simulink model "pend"  (R2018b)
settings: Solver=ode45  StartTime=0.0  StopTime=1.4  RelTol=1e-6
values from neighbouring files (symbols this model uses):
  g = 9.81    [plate_pend.m]
  J_zz = m_plate*(Lx^2+Ly^2)/3    (= 2.1087)    [plate_pend.m]
  Lx = 0.5    [parameters.m]    (also in plate_pend.m = 0.6)
  Ly = 0.3    [parameters.m]    (also in plate_pend.m)
  m_plate = rho*h*Lx*Ly    (= 9.36)    [parameters.m]    (also in plate_pend.m = 14.058)
libraries: cstblocks x1
settings Model: Creator=a.brugnoli  LastModifiedBy=a.brugnoli

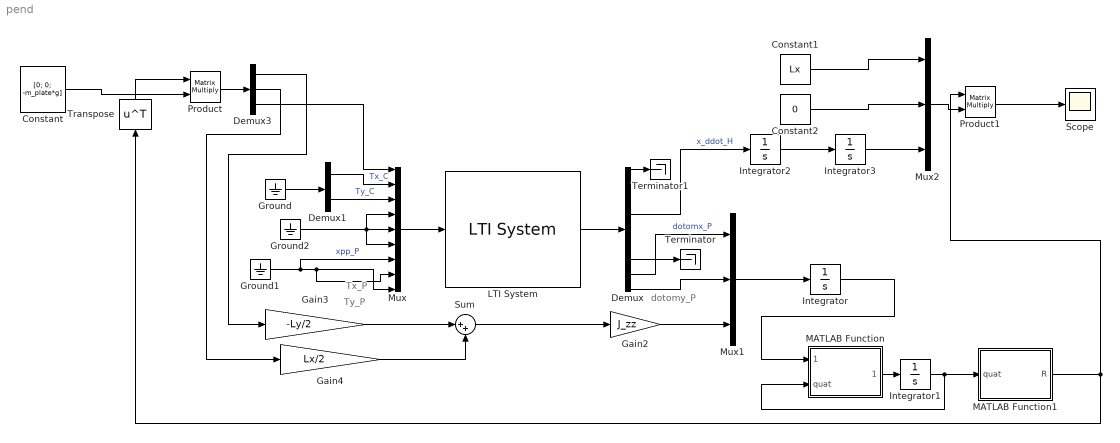
== system pend ==
  note: dotomy_P
  note: Ty_P
  note: Tx_P
  Constant : Constant  Value=[0; 0; -m_plate*g]  VectorParams1D=off
  Constant1 : Constant  Value=Lx
  Constant2 : Constant  Value=0
  Demux : Demux  Outputs=9
  Demux1 : Demux  Outputs=2
  Demux3 : Demux  Outputs=3
  Gain2 : Gain  Gain=J_zz
  Gain3 : Gain  Gain=-Ly/2
  Gain4 : Gain  Gain=Lx/2
  Ground : Ground
  Ground1 : Ground
  Ground2 : Ground
  Integrator : Integrator
  Integrator1 : Integrator  InitialCondition=[1, 0, 0, 0]
  Integrator2 : Integrator
  Integrator3 : Integrator
  LTI System : cstblocks/LTI System  sys=plate_pendulum  IC=[]
  MATLAB Function : MATLAB Function  TreatAsAtomicUnit=on
  MATLAB Function1 : MATLAB Function  TreatAsAtomicUnit=on
  Mux : Mux  Inputs=9
  Mux1 : Mux  Inputs=3
  Mux2 : Mux  Inputs=3
  Product : Product  Multiplication=Matrix(*)
  Product1 : Product  Multiplication=Matrix(*)
  Scope : Scope
  Sum : Sum  Inputs=|++
  Terminator : Terminator
  Terminator1 : Terminator
  Transpose : Math  Operator=transpose  SaturateOnIntegerOverflow=on
  wires:
  LTI System/1 -> Demux/1
  Mux/1 -> LTI System/1
  Ground/1 -> Demux1/1
  Demux1/2 -> Mux/3  "Ty_C"
  Demux1/1 -> Mux/2  "Tx_C"
  Gain2/1 -> Mux1/3
  Ground1/1 -> Mux/9, Mux/8, Mux/7  "xpp_P"
  Demux3/3 -> Mux/1
  Demux3/2 -> Gain4/1
  Demux3/1 -> Gain3/1
  Mux1/1 -> Integrator/1
  Integrator/1 -> MATLAB Function/1(omega)
  MATLAB Function/1(dt_quat) -> Integrator1/1
  Integrator1/1 -> MATLAB Function1/1(quat), MATLAB Function/2(quat)
  MATLAB Function1/1(R) -> Product1/1, Transpose/1
  Transpose/1 -> Product/1
  Constant/1 -> Product/2
  Product/1 -> Demux3/1
  Gain4/1 -> Sum/2
  Gain3/1 -> Sum/1
  Sum/1 -> Gain2/1
  Demux/9 -> Mux1/2
  Demux/8 -> Mux1/1  "dotomx_P"
  Demux/7 -> Terminator/1
  Demux/4 -> Integrator2/1  "x_ddot_H"
  Ground2/1 -> Mux/6, Mux/4, Mux/5
  Integrator2/1 -> Integrator3/1
  Integrator3/1 -> Mux2/3
  Constant2/1 -> Mux2/2
  Constant1/1 -> Mux2/1
  Mux2/1 -> Product1/2
  Product1/1 -> Scope/1
  Demux/1 -> Terminator1/1

== matlab function pend/MATLAB Function1 ==
  data: R output; quat input
function R = rot_mat(quat)

a = quat(1);
b = quat(2);
c = quat(3);
d = quat(4);


R = [2*a^2 + 2*b^2-1, 2*b*c - 2*b*a, 2*b*d + 2*a*c;
     2*b*c + 2*a*d, 2*a^2+2*c^2-1, 2*c*d - 2*a*b;
     2*b*d - 2*a*c, 2*c*d + 2*a*b, 2*a^2 + 2*d^2 - 1];

== matlab function pend/MATLAB Function ==
  data: omega input; dt_quat output; quat input
function dt_quat = quat_int(omega, quat)


omega_mat = [0, -omega(1), -omega(2), -omega(3);
             omega(1), 0, omega(3), -omega(2);
             omega(2), -omega(3), 0, omega(1);
             omega(3), omega(2), -omega(1), 0];

     
dt_quat = 0.5*omega_mat * quat;
